simulink library "Power_Ideal1Motor"  (R2018b)
settings: Solver=VariableStepAuto  StartTime=0.0  StopTime=10.0  RelTol=1e-3
libraries: fl_lib x6, nesl_utility x3, sm_lib x1
Description:
  | Component of Simscape Vehicle Templates Library
  | 
  | Copyright 2018-2020 The MathWorks, Inc.
settings Model: Creator=smiller  LastModifiedBy=smiller

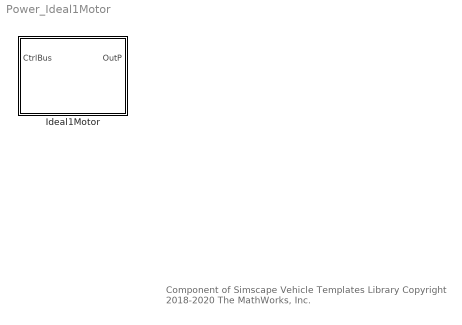
== system Power_Ideal1Motor ==
  note: Component of Simscape Vehicle Templates Library
      | Copyright 2018-2020 The MathWorks, Inc.
  Ideal1Motor : Subsystem  VariantControl=IdealOneMotor  mask(Single Ideal Motor){motor_ts_f=100, motor_ts_r=100}
      mask prompts: motor_ts_f "Front Motor Cutoff Frequency (Hz)"; motor_ts_r "Rear Motor Cutoff Frequency (Hz)"
      mask Display: image('sm_car_vehicle_power_ideal1motor_IMAGE.png');

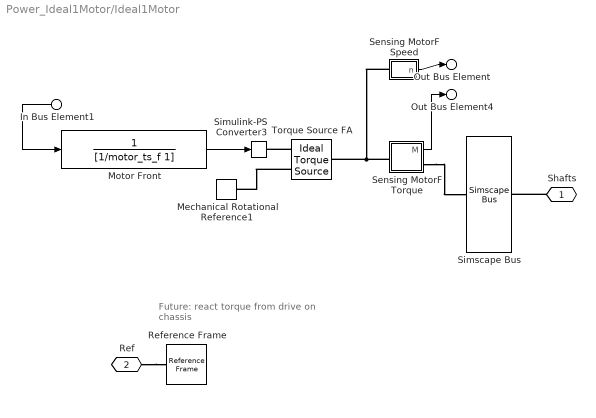
== system Power_Ideal1Motor/Ideal1Motor ==
  note: Future: react torque from
      | drive on chassis
  In Bus Element1 : Inport  PortName=CtrlBus  Element=MMotorFDemand
  Mechanical Rotational Reference1 : fl_lib/Mechanical/Rotational Elements/Mechanical Rotational Reference
  Motor Front : TransferFcn  Denominator=[1/motor_ts_f 1]
  Reference Frame : sm_lib/Frames and Transforms/Reference Frame
  Sensing MotorF Speed : Subsystem
  Sensing MotorF Torque : Subsystem
  Simscape Bus : SimscapeBus  HierarchyStrings=ShaftF
  Simulink-PS Converter3 : nesl_utility/Simulink-PS Converter  PhysicalDomain=network_engine_domain  SubClassName=ps_input  LeftPortType=input  RightPortType=output  PseudoPeriodic=off  Frequencies=[]  NoiseDistribution=none  NoiseParameters=[]  Unit=1  AffineConversion=off  FilteringAndDerivatives=provide  SimscapeFilterOrder=1  InputFilterTimeConstant=0.001  UdotUserProvided=0
  Torque Source FA : fl_lib/Mechanical/Mechanical Sources/Ideal Torque Source
  Shafts : PMIOPort  Side=Left
  Ref : PMIOPort  Port=2  Side=Right
  Out Bus Element : Outport  PortName=OutP  Element=nMotorF
  Out Bus Element4 : Outport  PortName=OutP  Element=MMotorF
  wires:
  Sensing MotorF Speed/1(n) -> Out Bus Element/1
  In Bus Element1/1 -> Motor Front/1
  Motor Front/1 -> Simulink-PS Converter3/1
  Sensing MotorF Torque/1(M) -> Out Bus Element4/1
  connections:
  Sensing MotorF Speed/LConn1 -- Sensing MotorF Torque/LConn1 -- Torque Source FA/LConn1
  Torque Source FA/RConn1 -- Simulink-PS Converter3/RConn1
  Torque Source FA/RConn2 -- Mechanical Rotational Reference1/LConn1
  Shafts/RConn1 -- Simscape Bus/RConn1
  Ref/RConn1 -- Reference Frame/RConn1
  Sensing MotorF Torque/RConn1 -- Simscape Bus/LConn1

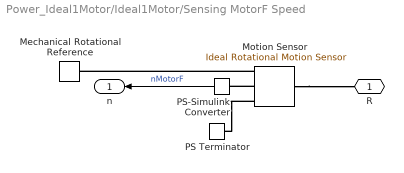
== system Power_Ideal1Motor/Ideal1Motor/Sensing MotorF Speed ==
  Mechanical Rotational Reference : fl_lib/Mechanical/Rotational Elements/Mechanical Rotational Reference
  Motion Sensor : fl_lib/Mechanical/Mechanical Sensors/Ideal Rotational Motion Sensor  offset=0 rad
  PS Terminator : fl_lib/Physical Signals/Sinks/PS Terminator
      settings: SourceProductName=Simscape
  PS-Simulink Converter : nesl_utility/PS-Simulink Converter  PhysicalDomain=network_engine_domain  SubClassName=ps_output  LeftPortType=input  RightPortType=output  PseudoPeriodic=off  Frequencies=[]  Unit=rad/s  AffineConversion=off
  R : PMIOPort  Side=Left
  n : Outport
  wires:
  PS-Simulink Converter/1 -> n/1  "nMotorF"
  connections:
  Motion Sensor/RConn2 -- PS-Simulink Converter/LConn1
  Motion Sensor/RConn3 -- PS Terminator/LConn1
  Motion Sensor/LConn1 -- R/RConn1
  Motion Sensor/RConn1 -- Mechanical Rotational Reference/LConn1

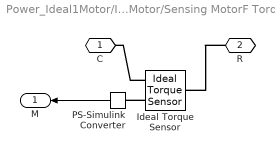
== system Power_Ideal1Motor/Ideal1Motor/Sensing MotorF Torque ==
  Ideal Torque Sensor : fl_lib/Mechanical/Mechanical Sensors/Ideal Torque Sensor
  PS-Simulink Converter : nesl_utility/PS-Simulink Converter  PhysicalDomain=network_engine_domain  SubClassName=ps_output  LeftPortType=input  RightPortType=output  PseudoPeriodic=off  Frequencies=[]  Unit=N*m  AffineConversion=off
  C : PMIOPort  Side=Right
  R : PMIOPort  Port=2  Side=Left
  M : Outport
  wires:
  PS-Simulink Converter/1 -> M/1
  connections:
  Ideal Torque Sensor/RConn2 -- PS-Simulink Converter/LConn1
  R/RConn1 -- Ideal Torque Sensor/LConn1
  Ideal Torque Sensor/RConn1 -- C/RConn1
